simulink model "testrig_BodyGeometry_Trailer"  (R2025b)
settings: Solver=VariableStepAuto  StartTime=0.0  StopTime=30  RelTol=1e-3  EnableMultiTasking=on
undefined symbols (not defined in the file): Visual, X, Y, Z
libraries: sm_lib x4, nesl_utility x2, BodyGeometry_Basic_Trailer x1, BodyGeometry_Box_Trailer x1, BodyLoad_Slosh_Pend3 x1, BodyGeometry_Tank_Trailer x1
Description:
  | Copyright 2021-2025 The MathWorks, Inc.
settings Model: Creator=smiller  LastModifiedBy=smiller
settings SolverCC: AlgebraicLoopSolver=TrustRegion
settings DataIOCC: LimitDataPoints=on  ReturnWorkspaceOutputs=off  SignalLoggingName=logsout_testrig_BodyGeometry_Trailer
settings OptimizationCC: ReuseModelBlockBuffer=off  LifeSpan=inf
settings DebuggingCC: UnconnectedInputMsg=warning  UnconnectedOutputMsg=warning  UnconnectedLineMsg=warning  AllowSymbolicDim=off  SFUnexpectedBacktrackingDiag=warning  SFNoUnconditionalDefaultTransitionDiag=warning  SFExecutionAtInitializationDiag=none  ArithmeticOperatorsInVariantConditions=warning
settings ModelReferenceCC: EnableRefExpFcnMdlSchedulingChecks=on
settings SFSimCC: SimUseLocalCustomCode=off  CustomCodeUndefinedFunction=UseInterfaceOnly
settings RTWCC: RTWUseLocalCustomCode=off  GPUComputeCapability=3.5  DLArmComputeVersion=19.05
settings CodeAppCC: StateflowObjectComments=on
settings GRTTargetCC: TargetLangStandard=C89/C90 (ANSI)
settings ConfigComp: CovMetricSettings=dw  CovSaveCumulativeToWorkspaceVar=on  CovSaveSingleToWorkspaceVar=on  CovExternalEMLEnable=off  CovSFcnEnable=off
settings SimscapeCC: SimscapeNominalValues="[{\"value\":\"10\",\"unit\":\"V\"},{\"value\":\"1\",\"unit\":\"A\"},{\"value\":\"10\",\"unit\":\"N*m\"},{\"value\":\"10\",\"unit\":\"bar\"},{\"value\":\"100\",\"unit\":\"kJ/kg\"},{\"value\":\"1\",\"unit\":\"kW\"},{\"value\":\"300\",\"unit\":\"K\"},{\"value\":\"100\",\"unit\":\"cm^3/s\"},{\"value\":\"1\",\"unit\":\"kN\"},{\"value\":\"1\",\"unit\":\"g/cm^3\"},{\"value\":\"1\",\"unit\":\"l\"},{\"value\":\"1\",\"unit\":\"cm^2\"},{\"value\":\"60\",\"unit\":\"Hz\"}]"  SimscapeLogType=all  SimscapeLogName=simlog_testrig_BodyGeometry_Trailer  SimscapeLogDataHistory=10000.0
settings ConfigurationSet: Description=SimMechanics 2G
settings ExplorerConfigSet: InternalSimMechanicsExplorerSettings="<ExplorerConfiguration><canonicalview>default</canonicalview><AnimationSetting><BasePlaybackSpeed>1.0</BasePlaybackSpeed><PlaybackSpeedFactor>4.0</PlaybackSpeedFactor></AnimationSetting><TilePanel><TileInfo><Tiles Columns=\"1\" Count=\"1\" Rows=\"1\"><Column Weight=\"1\"/><Row Weight=\"1\"/><Tile Height=\"1\" Width=\"1\" X=\"0\" Y=\"0\"/></Tiles></TileInfo><SceneInfo><SceneViewer><BGColor><R>1</R><G>1</G><B>1</B></BGColor><Camera><DoPerspective>off</DoPerspective><Position><X>13.4155182667225752</X><Y>2.28677307770006744</Y><Z>4.62010338736664927</Z></Position><Center><X>3.73535822442298659</X><Y>3.85693218623915524</Y><Z>2.80389459364715421</Z></Center><Up><X>-0.1819255686100896</X><Y>0.0156704114335161071</Y><Z>0.983187431617898677</Z></Up><ViewLimDist>1</ViewLimDist><YLim>6.28718702529015783</YLim><XLim>6.374240384101868</XLim></Camera></SceneViewer></SceneInfo></TilePanel><MechEditorPanel><Cameras/><GfxPanelCameraMap/><VideoCreator><PlaybackSpeedRatio>1.0</PlaybackSpeedRatio><FrameRate>30</FrameRate><VideoFormat>Motion JPEG AVI</VideoFormat><FrameSize>auto</FrameSize></VideoCreator></MechEditorPanel></ExplorerConfiguration>"

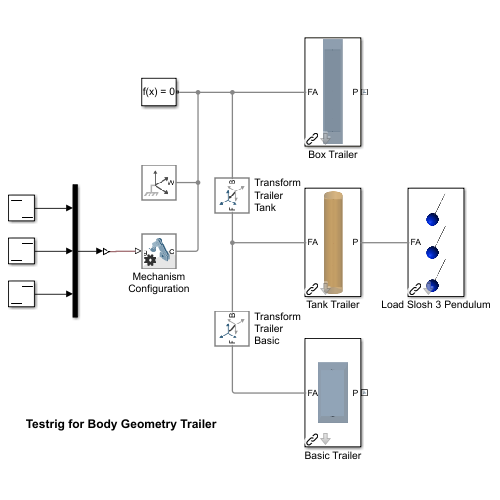
[thumbnail: Simulink's stored preview of the top-level diagram]
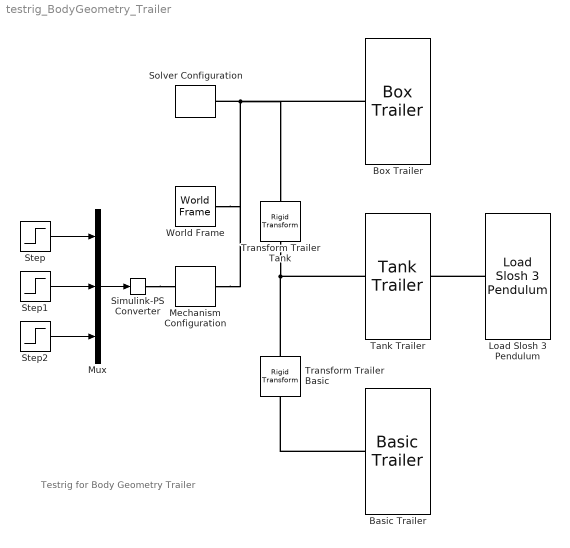
== system testrig_BodyGeometry_Trailer ==
  note: Testrig for Body Geometry Trailer
  Basic Trailer : BodyGeometry_Basic_Trailer/Basic Trailer  body_length=VDatabase.BodyGeometry.Basic_Trailer_Elula.xLength.Value  body_height=VDatabase.BodyGeometry.Basic_Trailer_Elula.xHeight.Value  body_width=VDatabase.BodyGeometry.Basic_Trailer_Elula.xWidth.Value  offset_ref=[0 0 0.4]  extr_data_emblem_f=Visual.emblem.data*0.2  extr_data_emblem_r=Visual.emblem.data*0.2  clr_body_geo_top=VDatabase.BodyGeometry.Basic_Trailer_Elula.Color.Value  opc_body_geo_top=Visual.body.opc  clr_emblem_f=VDatabase.BodyGeometry.Basic_Trailer_Elula.EmblemColor.Value  opc_emblem_f=Visual.emblem.opc  clr_emblem_r=VDatabase.BodyGeometry.Basic_Trailer_Elula.EmblemColor.Value  opc_emblem_r=Visual.emblem.opc
  Box Trailer : BodyGeometry_Box_Trailer/Box Trailer  VariantControl=Sedan  box_lwh=[13 2.5 2.7]  bed_lwh=[13 2.5 0.2]  bed_z=1.5  bed_box_xOffset=0  xReftoFront=10  extr_data_emblem_f=Visual.emblem.data*0.2  extr_data_emblem_r=Visual.emblem.data*0.2  clr_body_geo_top=[0.2 0.4 0.6]  opc_body_geo_top=1  clr_body_geo_left=[0.8 0.8 0.8]  opc_body_geo_left=1  clr_emblem_f=[1 1 1]  opc_emblem_f=Visual.emblem.opc  clr_emblem_r=[1 1 1]  opc_emblem_r=Visual.emblem.opc
  Load Slosh 3 Pendulum : BodyLoad_Slosh_Pend3/Load Slosh 3 Pendulum  refToPendCtr=[10-13/2 0 1.5+0.2+1.25+1]  pend_sep=3  damping_rx=0.1  damping_ry=0.1  pend_len=1  pend_mass=10
  Mechanism Configuration : sm_lib/Utilities/Mechanism Configuration  UniformGravity=TimeVarying  GravityVector=[0 0 -9.80665]  GravityVectorUnits=m/s^2  LinearizationDelta=0.001  JointModeTransitionNonlinearIterations=2
  Mux : Mux  Inputs=3
  Simulink-PS Converter : nesl_utility/Simulink-PS Converter  PhysicalDomain=network_engine_domain  SubClassName=ps_input  LeftPortType=input  RightPortType=output  PseudoPeriodic=off  Frequencies=[]  NoiseDistribution=none  NoiseParameters=[]  Unit=1  AffineConversion=off  FilteringAndDerivatives=provide  SimscapeFilterOrder=1  InputFilterTimeConstant=0.001  UdotUserProvided=0
  Solver Configuration : nesl_utility/Solver Configuration  PhysicalDomain=network_engine_domain  SubClassName=solver  LeftPortType=input  RightPortType=generic  Tones=[]  Harmonics=[]  SimulateNoise=off  Profile=off  UseLocalSampling=off  EnableSwitchedLinearOptims=on  FrequencyDomain=off  UseCCode=off  RelTol=0.001  AbsTol=1e-06  MinStep=1e-09  ToWorkspace=off  RevertToSquareIcSolve=off  NumHomotopyIterations=100  PhasorMode=off  PhasorModeNumHarmonics=1  ConsistencySolver=NEWTON_FTOL  IndexReductionMethod=DerivativeReplacement  DoDC=off  ResidualTolerance=1e-09  ConsistencyTolSource=GLOBAL  ConsistencyAbsTol=0.001  ConsistencyRelTol=0.001  ConsistencyTolFactor=0.001  UseLocalSolver=off  LocalSolverChoice=NE_BACKWARD_EULER_ADVANCER  ResolveIndetEquations=on  FunctionEvalNumThread=1  LocalSolverSampleTime=0.001  DoFixedCost=off  MaxNonlinIter=3  MaxModeIter=2  ComputeImpulses=off  ImpulseIterations=2  LinearAlgebra=Sparse  LinearAlgebraNumThread=0  EquationFormulation=NE_TIME_EF  DelaysMemoryBudget=1024  AutomaticFiltering=on  FilteringTimeConstant=0.001  PartitionStorageMethod=AS_NEEDED  PartitionMemoryBudget=1024  PartitionMethod=FAST  MultibodyUseLocalSolver=off  MultibodyLocalSolverChoice=ODE1  MultibodyLocalSolverSampleTime=0.001
  Step : Step  Time=5  After=-1  SampleTime=0
  Step1 : Step  Time=15  After=0.5  SampleTime=0
  Step2 : Step  Time=5  Before=-1  After=-0.5  SampleTime=0
  Tank Trailer : BodyGeometry_Tank_Trailer/Tank Trailer  VariantControl=Sedan  tank_len=13  tank_rad=1.25  bed_lwh=[13 2.5 0.2]  bed_z=1.5  bed_tank_xOffset=0  xReftoFront=10  extr_data_emblem_f=Visual.emblem.data*0.2  extr_data_emblem_r=Visual.emblem.data*0.2  clr_body_geo_top=[1 0.6 0]  opc_body_geo_top=Visual.body.opc  clr_body_geo_left=[0.8 0.8 0.8]  opc_body_geo_left=Visual.body.opc  clr_emblem_f=[1 1 1]  opc_emblem_f=Visual.emblem.opc  clr_emblem_r=[1 1 1]  opc_emblem_r=Visual.emblem.opc
  Transform Trailer Basic : sm_lib/Frames and Transforms/Rigid Transform  RotationMethod=None  FollAlignAxisA=+X  BaseAlignAxisA=+Y  FollAlignAxisB=+Y  BaseAlignAxisB=+Z  RotationStandardAxis=+Z  RotationAngle=0.0  RotationAngleUnits=deg  RotationArbitraryAxis=[0 0 1]  RotationSequenceAxes=FollowerAxes  RotationSequence=XYX  RotationSequenceAngles=[0 0 0]  RotationSequenceAnglesUnits=deg  RotationMatrix=[1 0 0; 0 1 0; 0 0 1]  Quaternion=[1 0 0 0]  TranslationMethod=Cartesian  TranslationCartesianOffset=[0 5 0]  TranslationCartesianOffsetUnits=m  TranslationStandardAxis=+Z  TranslationStandardOffset=0  TranslationStandardOffsetUnits=m  TranslationROffset=0  TranslationROffsetUnits=m  TranslationThetaOffset=0  TranslationThetaOffsetUnits=deg  TranslationZOffset=0  TranslationZOffsetUnits=m
  Transform Trailer Tank : sm_lib/Frames and Transforms/Rigid Transform  RotationMethod=None  FollAlignAxisA=+X  BaseAlignAxisA=+Y  FollAlignAxisB=+Y  BaseAlignAxisB=+Z  RotationStandardAxis=+Z  RotationAngle=0.0  RotationAngleUnits=deg  RotationArbitraryAxis=[0 0 1]  RotationSequenceAxes=FollowerAxes  RotationSequence=XYX  RotationSequenceAngles=[0 0 0]  RotationSequenceAnglesUnits=deg  RotationMatrix=[1 0 0; 0 1 0; 0 0 1]  Quaternion=[1 0 0 0]  TranslationMethod=Cartesian  TranslationCartesianOffset=[0 5 0]  TranslationCartesianOffsetUnits=m  TranslationStandardAxis=+Z  TranslationStandardOffset=0  TranslationStandardOffsetUnits=m  TranslationROffset=0  TranslationROffsetUnits=m  TranslationThetaOffset=0  TranslationThetaOffsetUnits=deg  TranslationZOffset=0  TranslationZOffsetUnits=m
  World Frame : sm_lib/Frames and Transforms/World Frame
  wires:
  Step/1 -> Mux/1
  Step1/1 -> Mux/2
  Step2/1 -> Mux/3
  Mux/1 -> Simulink-PS Converter/1
  connections:
  Mechanism Configuration/RConn1 -- World Frame/RConn1 -- Box Trailer/RConn1 -- Transform Trailer Tank/LConn1 -- Solver Configuration/RConn1
  Simulink-PS Converter/RConn1 -- Mechanism Configuration/LConn1
  Transform Trailer Tank/RConn1 -- Tank Trailer/RConn1 -- Transform Trailer Basic/LConn1
  Basic Trailer/RConn1 -- Transform Trailer Basic/RConn1
  Load Slosh 3 Pendulum/LConn1 -- Tank Trailer/LConn1
